simulink model "slo_distpipe"  (R2015b)
settings: Solver=FixedStepDiscrete  SolverMode=SingleTasking  StartTime=0.0  StopTime=10.0  RelTol=1e-3
libraries: simulink x2
settings Model: Creator=amatsumo  LastModifiedBy=amatsumo
settings DataIOCC: SaveFormat=Array  SignalLoggingSaveFormat=ModelDataLogs  SaveOutput=off  SignalLogging=off  SaveTime=off
settings OptimizationCC: BlockReduction=off  ConditionallyExecuteInputs=off  DefaultParameterBehavior=Inlined  ExpressionDepthLimit=2147483647
settings DebuggingCC: AlgebraicLoopMsg=error  UnderspecifiedInitializationDetection=Classic  MergeDetectMultiDrivingBlocksExec=none  SolverPrmCheckMsg=warning  InheritedTsInSrcMsg=none  SingleTaskRateTransMsg=error  FcnCallInpInsideContextMsg=UseLocalSettings  StateNameClashWarn=warning
settings HardwareCC: ProdBitPerPointer=32  ProdLargestAtomicFloat=None  ProdIntDivRoundTo=Undefined  ProdEndianess=Unspecified  ProdWordSize=32  ProdHWDeviceType=ASIC/FPGA->ASIC/FPGA  ProdEqTarget=off
settings GRTTargetCC: GeneratePreprocessorConditionals=Disable all  CombineOutputUpdateFcns=off  GRTInterface=on
settings ConfigComp: CovModelRefEnable=Off  CovSFcnEnable=off

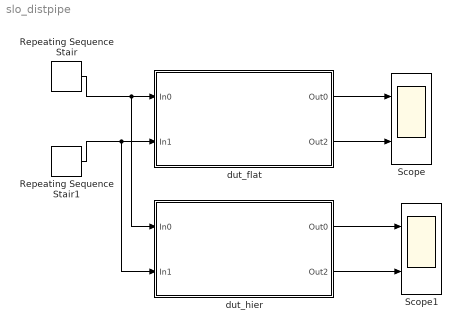
== system slo_distpipe ==
  Repeating Sequence Stair : simulink/Sources/Repeating Sequence Stair  OutValues=[1 2 3].'  tsamp=1  OutMin=[]  OutMax=[]  OutDataTypeStr=fixdt(1,8,0)  OutputDataTypeScalingMode=Specify via dialog  OutDataType=fixdt(1,8,0)  ConRadixGroup=Best Precision: Vector-wise  OutScaling=[]
  Repeating Sequence Stair1 : simulink/Sources/Repeating Sequence Stair  OutValues=[1 3 4 5].'  tsamp=1  OutMin=[]  OutMax=[]  OutDataTypeStr=fixdt(1,8,0)  OutputDataTypeScalingMode=Specify via dialog  OutDataType=fixdt(1,8,0)  ConRadixGroup=Best Precision: Vector-wise  OutScaling=[]
  Scope : Scope  NumInputPorts=2
  Scope1 : Scope  NumInputPorts=2
  dut_flat : Subsystem
  dut_hier : Subsystem
  wires:
  dut_flat/1(Out0) -> Scope/1
  Repeating Sequence Stair/1 -> dut_flat/1(In0), dut_hier/1(In0)
  Repeating Sequence Stair1/1 -> dut_flat/2(In1), dut_hier/2(In1)
  dut_flat/2(Out2) -> Scope/2
  dut_hier/1(Out0) -> Scope1/1
  dut_hier/2(Out2) -> Scope1/2

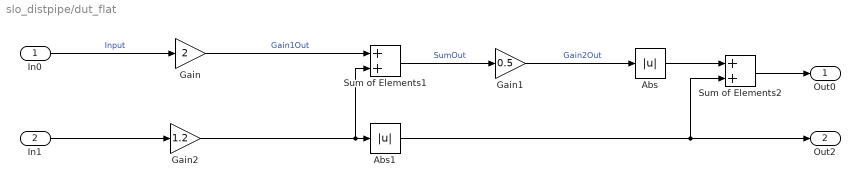
== system slo_distpipe/dut_flat ==
  In0 : Inport
  In1 : Inport  Port=2
  Abs : Abs
  Abs1 : Abs
  Gain : Gain  Gain=2  ParamDataTypeStr=fixdt(0,4,2)  OutDataTypeStr=Inherit: Same as input
  Gain1 : Gain  Gain=0.5  ParamMin=0.5  ParamMax=0.5  ParamDataTypeStr=fixdt(0,1,1)  OutDataTypeStr=Inherit: Same as input
  Gain2 : Gain  Gain=1.2  ParamDataTypeStr=fixdt(0,4,2)  OutDataTypeStr=Inherit: Same as input
  Sum of Elements1 : Sum  OutDataTypeStr=Inherit: Same as first input
  Sum of Elements2 : Sum  OutDataTypeStr=Inherit: Same as first input
  Out0 : Outport
  Out2 : Outport  Port=2
  wires:
  Sum of Elements2/1 -> Out0/1
  Abs/1 -> Sum of Elements2/1
  Abs1/1 -> Sum of Elements2/2, Out2/1
  In1/1 -> Gain2/1
  Gain2/1 -> Abs1/1, Sum of Elements1/2
  In0/1 -> Gain/1  "Input"
  Gain1/1 -> Abs/1  "Gain2Out"
  Sum of Elements1/1 -> Gain1/1  "SumOut"
  Gain/1 -> Sum of Elements1/1  "Gain1Out"

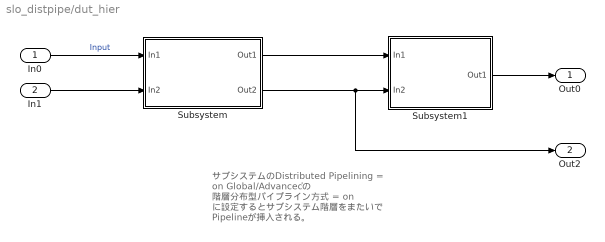
== system slo_distpipe/dut_hier ==
  note: サブシステムのDistributed Pipelining = on
      | Global/Advancedの
      | 階層分布型パイプライン方式 = on
      | に設定するとサブシステム階層をまたいで
      | Pipelineが挿入される。
  In0 : Inport
  In1 : Inport  Port=2
  Subsystem : Subsystem
  Subsystem1 : Subsystem
  Out0 : Outport
  Out2 : Outport  Port=2
  wires:
  Subsystem/1(Out1) -> Subsystem1/1(In1)
  In0/1 -> Subsystem/1(In1)  "Input"
  In1/1 -> Subsystem/2(In2)
  Subsystem/2(Out2) -> Out2/1, Subsystem1/2(In2)
  Subsystem1/1(Out1) -> Out0/1

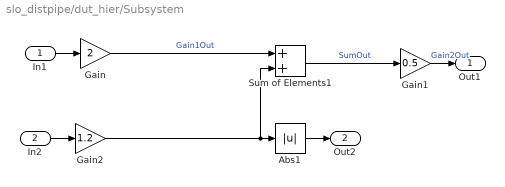
== system slo_distpipe/dut_hier/Subsystem ==
  In1 : Inport
  In2 : Inport  Port=2
  Abs1 : Abs
  Gain : Gain  Gain=2  ParamDataTypeStr=fixdt(0,4,2)  OutDataTypeStr=Inherit: Same as input
  Gain1 : Gain  Gain=0.5  ParamMin=0.5  ParamMax=0.5  ParamDataTypeStr=fixdt(0,1,1)  OutDataTypeStr=Inherit: Same as input
  Gain2 : Gain  Gain=1.2  ParamDataTypeStr=fixdt(0,4,2)  OutDataTypeStr=Inherit: Same as input
  Sum of Elements1 : Sum  OutDataTypeStr=Inherit: Same as first input
  Out1 : Outport
  Out2 : Outport  Port=2
  wires:
  Gain/1 -> Sum of Elements1/1  "Gain1Out"
  Sum of Elements1/1 -> Gain1/1  "SumOut"
  Gain2/1 -> Sum of Elements1/2, Abs1/1
  In1/1 -> Gain/1
  Gain1/1 -> Out1/1  "Gain2Out"
  Abs1/1 -> Out2/1
  In2/1 -> Gain2/1

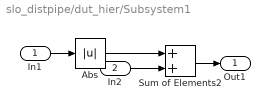
== system slo_distpipe/dut_hier/Subsystem1 ==
  In1 : Inport
  In2 : Inport  Port=2
  Abs : Abs
  Sum of Elements2 : Sum  OutDataTypeStr=Inherit: Same as first input
  Out1 : Outport
  wires:
  Abs/1 -> Sum of Elements2/1
  In2/1 -> Sum of Elements2/2
  In1/1 -> Abs/1
  Sum of Elements2/1 -> Out1/1
